simulink model "Magnetometer"  (R2021b)
settings: Solver=VariableStepAuto  StartTime=0.0  StopTime=500  RelTol=1e-3
model workspace (MAT data in the model file):
  K = 1
settings Model: Creator=kathe  LastModifiedBy=kathe

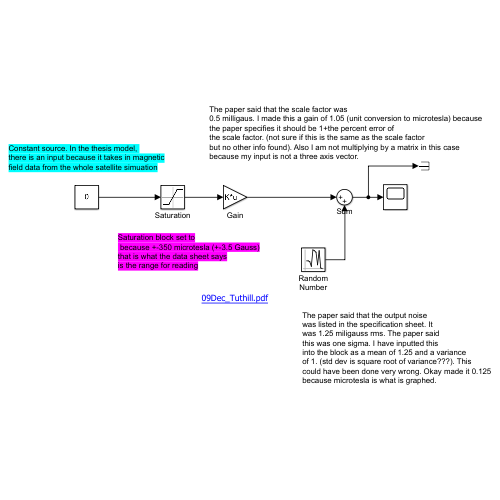
[thumbnail: Simulink's stored preview of the top-level diagram]
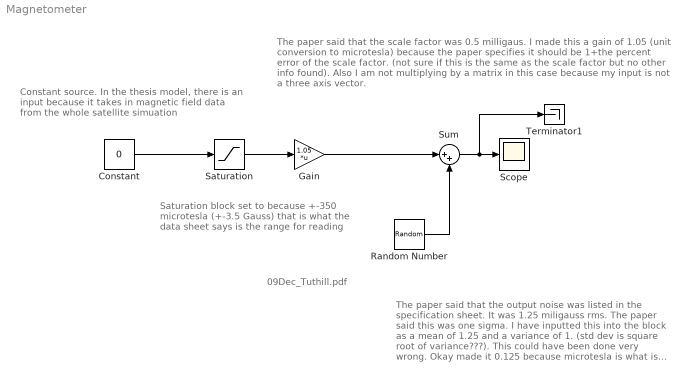
== system Magnetometer ==
  note: The paper said that the scale factor was
      | 0.5 milligaus. I made this a gain of 1.05 (unit conversion to microtesla) because
      | the paper specifies it should be 1+the percent error of
      | the scale factor. (not sure if this is the same as the scale factor
      | but no other info found). Also I am not multiplying by a matrix in this case
      | because my input is not a three axis vector.
  note: The paper said that the output noise
      | was listed in the specification sheet. It
      | was 1.25 miligauss rms. The paper said
      | this was one sigma. I have inputted this
      | into the block as a mean of 1.25 and a variance
      | of 1. (std dev is square root of variance???). This
      | could have been done very wrong. Okay made it 0.125
      | because microtesla is what is graphed.
  note: Saturation block set to
      | because +-350 microtesla (+-3.5 Gauss)
      | that is what the data sheet says
      | is the range for reading
  note: Constant source. In the thesis model,
      | there is an input because it takes in magnetic
      | field data from the whole satellite simuation
  note: 09Dec_Tuthill.pdf
  Constant : Constant  Value=0
  Gain : Gain  Gain=1.05  Multiplication=Matrix(K*u)
  Random Number : RandomNumber  Mean=0.125  SampleTime=0.1
  Saturation : Saturate  UpperLimit=350  LowerLimit=-350
  Scope : Scope
  Sum : Sum  Inputs=|++
  Terminator1 : Terminator
  wires:
  Constant/1 -> Saturation/1
  Saturation/1 -> Gain/1
  Gain/1 -> Sum/1
  Sum/1 -> Scope/1, Terminator1/1
  Random Number/1 -> Sum/2
